simulink model "ClosedLoopSys_SFunc"  (R2025b)
settings: Solver=FixedStepAuto  StartTime=0.00  StopTime=10  FixedStep=Ts  RelTol=1e-5  EnableMultiTasking=on
undefined symbols (not defined in the file or in its folder): DAC_lim_u, Discrete, l, N, nu, nx, par, Q, q, QN, Time, Ts, X0, x0
libraries: ctrlSharedLib x1
settings Model: Creator=bjones  LastModifiedBy=leeta
settings SolverCC: AlgebraicLoopSolver=TrustRegion
settings DataIOCC: SaveFormat=Array  SignalLoggingSaveFormat=ModelDataLogs  ReturnWorkspaceOutputs=off
settings OptimizationCC: BlockReduction=off  BooleanDataType=off  ExpressionDepthLimit=2147483647.0  LifeSpan=inf
settings DebuggingCC: SaveWithParameterizedLinksMsg=none  MergeDetectMultiDrivingBlocksExec=none  SignalResolutionControl=TryResolveAllWithWarning  MultiTaskDSMMsg=warning  MultiTaskCondExecSysMsg=none  FcnCallInpInsideContextMsg=warning  UnconnectedInputMsg=warning  UnconnectedOutputMsg=warning  UnconnectedLineMsg=warning  StateNameClashWarn=warning  SFUnexpectedBacktrackingDiag=warning  SFNoUnconditionalDefaultTransitionDiag=warning  SFExecutionAtInitializationDiag=none  ArithmeticOperatorsInVariantConditions=warning
settings HardwareCC: ProdBitPerPointer=32.0  ProdBitPerSizeT=32.0  ProdBitPerPtrDiffT=32.0  ProdLargestAtomicFloat=None  ProdIntDivRoundTo=Undefined  ProdEndianess=Unspecified  ProdWordSize=32.0  ProdHWDeviceType=32-bit Generic  TargetUnknown=on
settings ModelReferenceCC: EnableRefExpFcnMdlSchedulingChecks=on  PropagateSignalLabelsOutOfModel=off
settings SFSimCC: SimUseLocalCustomCode=off  CustomCodeUndefinedFunction=UseInterfaceOnly
settings RTWCC: RTWUseLocalCustomCode=off  GPUComputeCapability=3.5
settings CodeAppCC: StateflowObjectComments=on
settings GRTTargetCC: TargetLangStandard=C89/C90 (ANSI)  CombineOutputUpdateFcns=off  GRTInterface=on
settings ConfigComp: CovMetricSettings=dw  CovSaveCumulativeToWorkspaceVar=on  CovSaveSingleToWorkspaceVar=on  CovExternalEMLEnable=off  CovSFcnEnable=off

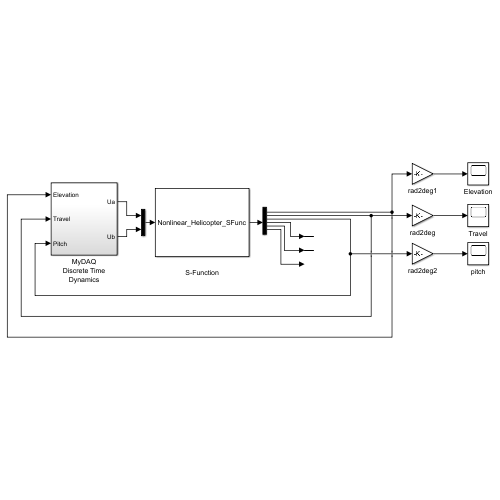
[thumbnail: Simulink's stored preview of the top-level diagram]
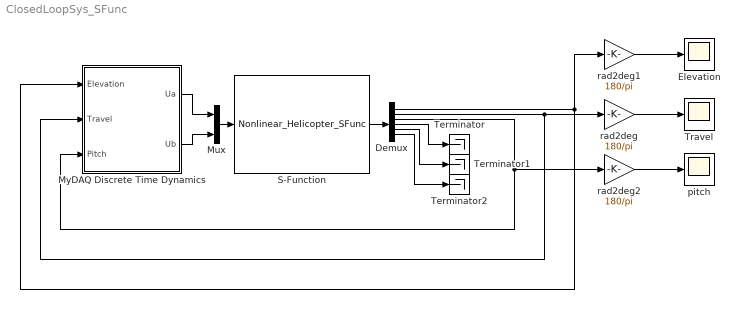
== system ClosedLoopSys_SFunc ==
  " S-Function" : S-Function  FunctionName=Nonlinear_Helicopter_SFunc  Parameters=par,X0  SFunctionDeploymentMode=off  EnableBusSupport=off
  Demux : Demux  Outputs=6
  Elevation : Scope
      settings: TimeSpan=60  ActiveDisplayYMinimum=-50  ActiveDisplayYMaximum=30  DataLoggingVariableName=elev
  Mux : Mux  Inputs=2
  MyDAQ Discrete Time Dynamics : Subsystem
  Terminator : Terminator
  Terminator1 : Terminator
  Terminator2 : Terminator
  Travel : Scope
      settings: TimeSpan=60  ActiveDisplayYMinimum=-150  ActiveDisplayYMaximum=300  DataLoggingVariableName=trav
  pitch : Scope
      settings: TimeSpan=60  ActiveDisplayYMinimum=-25  ActiveDisplayYMaximum=20  DataLoggingVariableName=pitch
  rad2deg : Gain  Gain=180/pi  SaturateOnIntegerOverflow=on  OutDataTypeStr=Inherit: Same as input  ParamDataTypeStr=Inherit: Same as input
  rad2deg1 : Gain  Gain=180/pi  SaturateOnIntegerOverflow=on  OutDataTypeStr=Inherit: Same as input  ParamDataTypeStr=Inherit: Same as input
  rad2deg2 : Gain  Gain=180/pi  SaturateOnIntegerOverflow=on  OutDataTypeStr=Inherit: Same as input  ParamDataTypeStr=Inherit: Same as input
  wires:
  rad2deg/1 -> Travel/1
  rad2deg1/1 -> Elevation/1
  Demux/2 -> MyDAQ Discrete Time Dynamics/2(Travel), rad2deg/1
  Demux/1 -> rad2deg1/1, MyDAQ Discrete Time Dynamics/1(Elevation)
  rad2deg2/1 -> pitch/1
  Demux/3 -> MyDAQ Discrete Time Dynamics/3(Pitch), rad2deg2/1
  MyDAQ Discrete Time Dynamics/1(Ua) -> Mux/1
  MyDAQ Discrete Time Dynamics/2(Ub) -> Mux/2
  Mux/1 -> " S-Function"/1
  " S-Function"/1 -> Demux/1
  Demux/4 -> Terminator/1
  Demux/5 -> Terminator1/1
  Demux/6 -> Terminator2/1

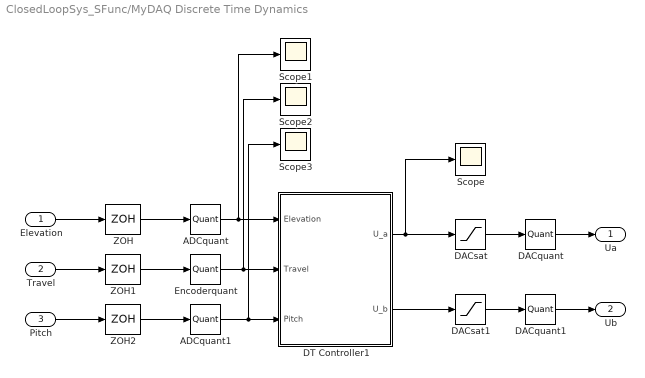
== system ClosedLoopSys_SFunc/MyDAQ Discrete Time Dynamics ==
  Elevation : Inport
  Travel : Inport  Port=2
  Pitch : Inport  Port=3
  ADCquant : Quantizer  QuantizationInterval=ADC_Vres
  ADCquant1 : Quantizer  QuantizationInterval=ADC_Vres
  DACquant : Quantizer  QuantizationInterval=DAC_Vres
  DACquant1 : Quantizer  QuantizationInterval=DAC_Vres
  DACsat : Saturate  UpperLimit=DAC_lim_u  LowerLimit=-DAC_lim_u
  DACsat1 : Saturate  UpperLimit=DAC_lim_u  LowerLimit=-DAC_lim_u
  DT Controller1 : Subsystem
  Encoderquant : Quantizer  QuantizationInterval=Encoder_res
  Scope{,1..3} (4 alike) : Scope
      Scope settings: ActiveDisplayYMinimum=-1  ActiveDisplayYMaximum=1
      Scope1 settings: ActiveDisplayYMinimum=-0.1017  ActiveDisplayYMaximum=0.78714  DataLoggingVariableName=ScopeData2
      Scope2 settings: ActiveDisplayYMinimum=-1  ActiveDisplayYMaximum=1
      Scope3 settings: ActiveDisplayYMinimum=-1  ActiveDisplayYMaximum=1  DataLoggingVariableName=ScopeData2
  ZOH : ZeroOrderHold  SampleTime=Ts
  ZOH1 : ZeroOrderHold  SampleTime=Ts
  ZOH2 : ZeroOrderHold  SampleTime=Ts
  Ua : Outport
  Ub : Outport  Port=2
  wires:
  Elevation/1 -> ZOH/1
  Travel/1 -> ZOH1/1
  DACquant/1 -> Ua/1
  DACquant1/1 -> Ub/1
  DT Controller1/1(U_a) -> Scope/1, DACsat/1
  DACsat/1 -> DACquant/1
  DT Controller1/2(U_b) -> DACsat1/1
  DACsat1/1 -> DACquant1/1
  ZOH1/1 -> Encoderquant/1
  ZOH/1 -> ADCquant/1
  Pitch/1 -> ZOH2/1
  ZOH2/1 -> ADCquant1/1
  ADCquant/1 -> Scope1/1, DT Controller1/1(Elevation)
  ADCquant1/1 -> Scope3/1, DT Controller1/3(Pitch)
  Encoderquant/1 -> Scope2/1, DT Controller1/2(Travel)

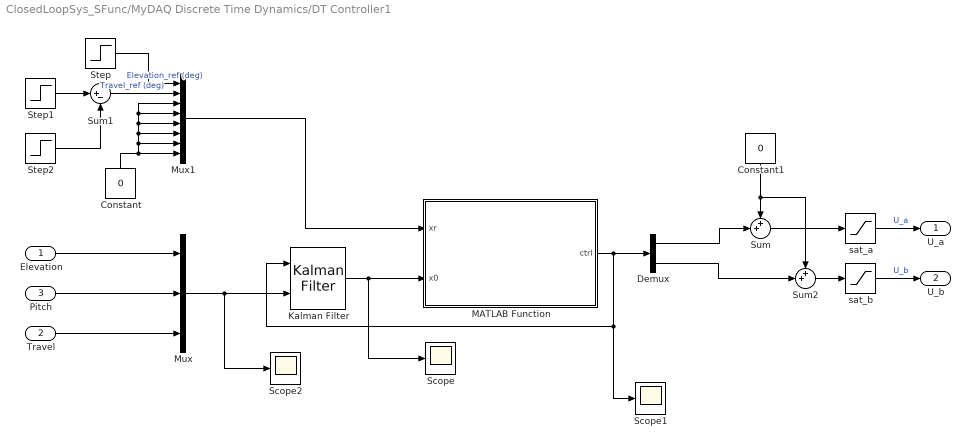
== system ClosedLoopSys_SFunc/MyDAQ Discrete Time Dynamics/DT Controller1 ==
  Elevation : Inport
  Travel : Inport  Port=2
  Pitch : Inport  Port=3
  Constant : Constant  Value=0
  Constant1 : Constant  Value=0
  Demux : Demux  Outputs=2
  Kalman Filter : ctrlSharedLib/Kalman Filter  TimeDomain=Discrete-Time  UseCurrentEstimator=on  ModelSource=LTI State-Space Variable  ModelSourceVariable=sysdt_comb  A=0.95  B=1  C=1  D=0  NumberOfStates=1  NumberOfInputs=1  NumberOfOutputs=1  InitialEstimateSource=Dialog  X0=x0  P0=10  UseK=off  UseGH=off  NumberOfProcessNoiseInputs=1  G=1  TimeInvariantG=on  H=0  TimeInvariantH=on  Q=0.05  TimeInvariantQ=on  R=1  TimeInvariantR=on  N=0  TimeInvariantN=on  AddInputPort=on  AddEnablePort=off  OutputEstimatedY=off  OutputP=off  Ts=-1
  MATLAB Function : MATLAB Function  TreatAsAtomicUnit=on
  Mux : Mux  Inputs=3
  Mux1 : Mux  Inputs=8
  Scope : Scope
      settings: ActiveDisplayYMinimum=-2.4396283803217269  ActiveDisplayYMaximum=1.6155430663981798  DataLoggingVariableName=ScopeData3
  Scope1 : Scope
      settings: ActiveDisplayYMinimum=-1  ActiveDisplayYMaximum=1  DataLoggingVariableName=ScopeData4
  Scope2 : Scope
      settings: ActiveDisplayYMinimum=-2.0543672469917391  ActiveDisplayYMaximum=1.1142569878492721  DataLoggingVariableName=ScopeData3
  Step : Step  Time=0  Before=x0(1)  After=0  SampleTime=Ts
  Step1 : Step  Time=x0(2)  After=0  SampleTime=Ts
  Step2 : Step  Time=0  Before=x0(3)  After=0  SampleTime=Ts
  Sum : Sum  Inputs=++|
  Sum1 : Sum  Inputs=|+-
  Sum2 : Sum  Inputs=++|
  sat_a : Saturate  UpperLimit=DAC_lim_u  LowerLimit=-DAC_lim_u
  sat_b : Saturate  UpperLimit=DAC_lim_u  LowerLimit=-DAC_lim_u
  U_a : Outport
  U_b : Outport  Port=2
  wires:
  Step1/1 -> Sum1/1
  Step2/1 -> Sum1/2
  sat_b/1 -> U_b/1  "U_b"
  sat_a/1 -> U_a/1  "U_a"
  Step/1 -> Mux1/1  "Elevation_ref (deg)"
  Sum1/1 -> Mux1/2  "Travel_ref (deg)"
  Elevation/1 -> Mux/1
  Pitch/1 -> Mux/2
  Travel/1 -> Mux/3
  Mux/1 -> Scope2/1, Kalman Filter/2
  Kalman Filter/1 -> Scope/1, MATLAB Function/2(x0)
  MATLAB Function/1(ctrl) -> Scope1/1, Kalman Filter/1, Demux/1
  Constant/1 -> Mux1/8, Mux1/6, Mux1/4, Mux1/3, Mux1/5, Mux1/7
  Mux1/1 -> MATLAB Function/1(xr)
  Demux/1 -> Sum/2
  Demux/2 -> Sum2/2
  Sum/1 -> sat_a/1
  Sum2/1 -> sat_b/1
  Constant1/1 -> Sum2/1, Sum/1

== matlab function ClosedLoopSys_SFunc/MyDAQ Discrete Time Dynamics/DT Controller1/MATLAB Function ==
  data: xr input double size=nx; x0 input double size=nx; ctrl output double size=nu; l parameter; u parameter; q parameter; Q parameter; QN parameter; nx parameter; nu parameter; N parameter
function ctrl = mpc_step(xr, x0, l, u, q, Q, QN, nx, nu, N)

    coder.extrinsic('emosqp')
    % Update OSQP problem
    % Update initial state

    l(1:nx) = -x0;
    u(1:nx) = -x0;
    % l(1:nx) = -(x0-xfe);
    % u(1:nx) = -(x0-xfe);

    % Update cost for variable xr
    q = [repmat(-Q*xr, N, 1); -QN*xr; zeros(N*nu, 1)];

    emosqp('update_bounds', l, u);
    emosqp('update_lin_cost', q);

    [x, ~, ~, ~, ~] = emosqp('solve'); 

    ctrl = x((N+1)*nx+1:(N+1)*nx+nu);
    % ctrl(1) = ctrl(1) + U_e;
    % ctrl(2) = ctrl(2) + U_e;
end
